simulink model "Mob_Cob_sim"  (R2023b)
settings: Solver=VariableStepAuto  StartTime=0.0  StopTime=5  MinStep=1e-5  RelTol=1e-2
values from neighbouring files (symbols this model uses):
  Mob_Cob = SerialLink(links,'name','Mobile_Cobot')    [Mob_Cob_plots.m]    (also in Omron_Mob_Cob.m; Omron_Mobile_Cobot.m; Updated_SCM_mobile_cobot_kinematics_no_dummy_frames.m; testing.m)
  q1 = ones(1,9)    [testing.m]
  q2 = ones(1,27)    [testing.m]
undefined symbols (not defined in the file or in its folder): coriolis, p560
libraries: roblocks x8
settings Model: Creator=jehuy  LastModifiedBy=kangwang

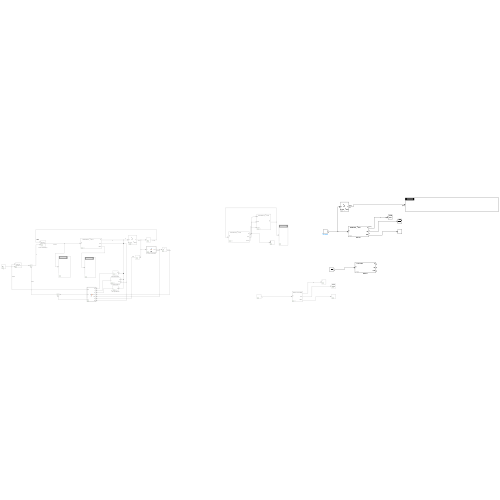
[thumbnail: Simulink's stored preview of the top-level diagram]
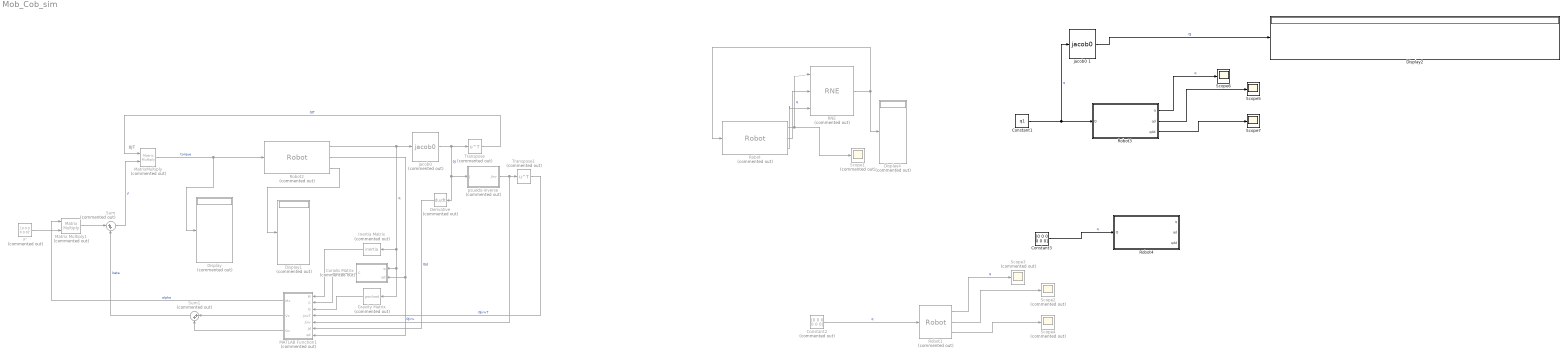
== system Mob_Cob_sim ==
  note: 0JT
  Constant1 : Constant  Value=q1
  Constant2 : Constant  Commented=on  Value=[0 0 0 0 0 0]
  Constant3 : Constant  Value=[0 0 0 0 0 0]
  Coriolis Matrix : Subsystem  Commented=on  mask{robot=Mob_Cob}
  Derivative : Derivative  Commented=on
  Display : Display  Commented=on
  Display1 : Display  Commented=on
  Display2 : Display
  Display4 : Display  Commented=on
  F' : Constant  Commented=on  Value=[0 0 0 0 0 0]'
  Gravity Matrix : roblocks/Arm/gravload  Commented=on  robot=Mob_Cob
  Inertia Matrix : roblocks/Arm/inertia  Commented=on  robot=Mob_Cob
  MATLAB Function1 : MATLAB Function  Commented=on  TreatAsAtomicUnit=on
  Matrix Multiply1 : Product  Commented=on  Multiplication=Matrix(*)
  MatrixMultiply : Product  Commented=on  Multiplication=Matrix(*)
  RNE : roblocks/Arm/RNE  Commented=on  robot=Mob_Cob.nofriction  grav=[0 0 9.81]
  Robot : roblocks/Arm/Robot  Commented=on  robot=Mob_Cob.nofriction  q0=[1 1 1 1 1 1 1 1 1]
      link override Integrator: InitialCondition=0
      link override Integrator1: InitialCondition=[1 1 1 1 1 1 1 1 1]
      link override S-Function: Parameters=robot
  Robot1 : roblocks/Arm/Robot  Commented=on  robot=p560.nofriction  q0=[0 0 0 0 0 0]
      link override Integrator1: InitialCondition=[0 0 0 0 0 0]
  Robot2 : roblocks/Arm/Robot  Commented=on  robot=Mob_Cob.nofriction  q0=[1 1 1 1 1 1 1 1 1]
      link override Integrator: InitialCondition=0
      link override Integrator1: InitialCondition=[1 1 1 1 1 1 1 1 1]
      link override S-Function: Parameters=robot
  Robot3 : Subsystem  AncestorBlock=roblocks/Arm/Robot  mask{robot=Mob_Cob.nofriction, q0=q1}
      mask prompts: robot "Robot object"; q0 "Initial state"
      mask help: Rigid-body dynamic model of robot.
      mask init:
      | if isa(robot, 'SerialLink')
      |     rname = robot.name;
      |     %fprintf('**robot name is %s\n', rname);
      | else
      |     rname = '';
      |     n = 0
      | end
      mask Help:
      | Simulates the forward (direct) rigid-body dynamics of the robot described
      | by the given robot object.  For given applied joint torque/force it computes
      | the instaneous joint coordinates, velocities and acclerations.
      | 
      | 
      | <b>Parameters::</b>
      | 
      | robot (SerialLink) a dynamic model of an N-link serial link manipulator
      | q0 (1xN)  Initial joint coordinates
      | 
      | <b>Inputs::</b>
      | 
      | Q (1xN) the generalized joint force (torque or force) required to achieve
      | the motion state (q, qd, qdd).
      | 
      | <b>Outputs::</b>
      | 
      | q (1xN) joint coordinates
      | qd (1xN) joint coordinate velocity
      | qdd (1xN) joint coordinate acceleration
      | 
      | 
      | <b>Notes::</b>
      | 
      | - Required to simulate robot rigid body motion.
      | - Implemented using the recursive Newton-Euler scheme (RNE).
      | - A wrapper for the Toolbox method accel() which in turn depends on the
      |   method rne().
      mask Display:
      | port_label('input', 1, 'Q')
      | port_label('output', 1, 'q')
      | port_label('output', 2, 'qd')
      | port_label('output', 3, 'qdd')
      | text(0.1, 0.9,  rname, 'horizontalAlignment', 'left')
  Robot4 : Subsystem  AncestorBlock=roblocks/Arm/Robot  mask{robot=p560, q0=q1}
      mask prompts: robot "Robot object"; q0 "Initial state"
      mask help: Rigid-body dynamic model of robot.
      mask init:
      | if isa(robot, 'SerialLink')
      |     rname = robot.name;
      |     %fprintf('**robot name is %s\n', rname);
      | else
      |     rname = '';
      |     n = 0
      | end
      mask Help:
      | Simulates the forward (direct) rigid-body dynamics of the robot described
      | by the given robot object.  For given applied joint torque/force it computes
      | the instaneous joint coordinates, velocities and acclerations.
      | 
      | 
      | <b>Parameters::</b>
      | 
      | robot (SerialLink) a dynamic model of an N-link serial link manipulator
      | q0 (1xN)  Initial joint coordinates
      | 
      | <b>Inputs::</b>
      | 
      | Q (1xN) the generalized joint force (torque or force) required to achieve
      | the motion state (q, qd, qdd).
      | 
      | <b>Outputs::</b>
      | 
      | q (1xN) joint coordinates
      | qd (1xN) joint coordinate velocity
      | qdd (1xN) joint coordinate acceleration
      | 
      | 
      | <b>Notes::</b>
      | 
      | - Required to simulate robot rigid body motion.
      | - Implemented using the recursive Newton-Euler scheme (RNE).
      | - A wrapper for the Toolbox method accel() which in turn depends on the
      |   method rne().
      mask Display:
      | port_label('input', 1, 'Q')
      | port_label('output', 1, 'q')
      | port_label('output', 2, 'qd')
      | port_label('output', 3, 'qdd')
      | text(0.1, 0.9,  rname, 'horizontalAlignment', 'left')
  Scope{1..4} (4 alike) : Scope  Commented=on
  Scope5 : Scope
  Scope6 : Scope
  Scope7 : Scope
  Sum : Sum  Commented=on  Inputs=|++
  Sum1 : Sum  Commented=on  Inputs=|++
  Transpose : Math  Commented=on  Operator=transpose
  Transpose1 : Math  Commented=on  Operator=transpose
  "jacob0 " : roblocks/Arm/jacob0   Commented=on  robot=Mob_Cob
  jacob0 1 : roblocks/Arm/jacob0   robot=Mob_Cob
  psuedo-inverse : MATLAB Function  Commented=on  TreatAsAtomicUnit=on
  wires:
  "jacob0 "/1 -> psuedo-inverse/1(J), Derivative/1, Transpose/1  "0J"
  psuedo-inverse/1(Jinv) -> MATLAB Function1/5(Jinv), Transpose1/1  "0Jinv"
  Transpose1/1 -> MATLAB Function1/4(JinvT)  "0JinvT"
  Transpose/1 -> MatrixMultiply/1  "0JT"
  Inertia Matrix/1 -> MATLAB Function1/1(M)
  Coriolis Matrix/1(C) -> MATLAB Function1/2(C)
  Derivative/1 -> MATLAB Function1/6(Jd)  "0Jd"
  MATLAB Function1/2(Vx) -> Sum1/1
  MATLAB Function1/3(Gx) -> Sum1/2
  Gravity Matrix/1 -> MATLAB Function1/3(G)
  Robot2/1 -> Gravity Matrix/1, Coriolis Matrix/1(q), Inertia Matrix/1, "jacob0 "/1  "q"
  F'/1 -> Matrix Multiply1/2
  MATLAB Function1/1(Mx) -> Matrix Multiply1/1  "alpha"
  Matrix Multiply1/1 -> Sum/1
  Sum1/1 -> Sum/2  "beta"
  Sum/1 -> MatrixMultiply/2  "F"
  MatrixMultiply/1 -> Robot2/1, Display/1  "torque"
  Constant2/1 -> Robot1/1  "q"
  Robot1/2 -> Scope2/1
  Robot1/1 -> Scope3/1  "q"
  Robot1/3 -> Scope4/1
  Robot/1 -> RNE/1, Scope1/1  "q"
  Robot2/2 -> MATLAB Function1/7(qd), Coriolis Matrix/2(qd)
  Robot2/3 -> Display1/1
  Robot/3 -> RNE/3
  Robot/2 -> RNE/2
  RNE/1 -> Display4/1, Robot/1
  Constant1/1 -> jacob0 1/1, Robot3/1(Q)  "q"
  Robot3/1(q) -> Scope6/1  "q"
  Robot3/2(qd) -> Scope5/1
  Robot3/3(qdd) -> Scope7/1
  jacob0 1/1 -> Display2/1  "0J"
  Constant3/1 -> Robot4/1(Q)  "q"

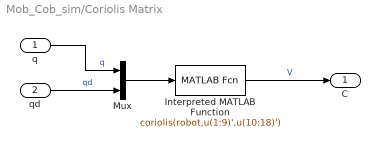
== system Mob_Cob_sim/Coriolis Matrix ==
  q : Inport
  qd : Inport  Port=2
  Interpreted MATLAB Function : MATLABFcn  MATLABFcn=coriolis(robot,u(1:9)',u(10:18)')  Output1D=off
  Mux : Mux  Inputs=2
  C : Outport
  wires:
  Mux/1 -> Interpreted MATLAB Function/1
  q/1 -> Mux/1  "q"
  qd/1 -> Mux/2  "qd"
  Interpreted MATLAB Function/1 -> C/1  "V"

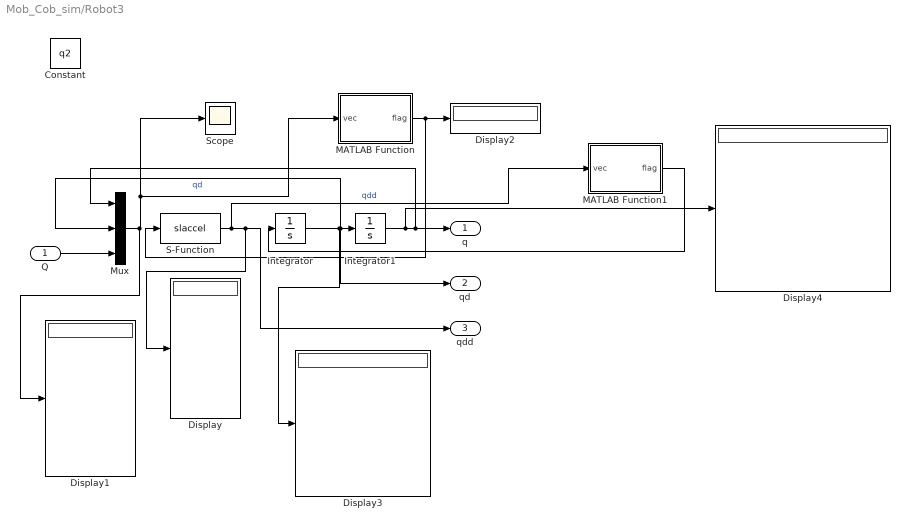
== system Mob_Cob_sim/Robot3 ==
  Q : Inport
  Constant : Constant  Value=q2
  Display{,1..4} (5 alike) : Display
  Integrator : Integrator
  Integrator1 : Integrator  InitialCondition=q1
  MATLAB Function : MATLAB Function  TreatAsAtomicUnit=on
  MATLAB Function1 : MATLAB Function  TreatAsAtomicUnit=on
  Mux : Mux  Inputs=3
  S-Function : S-Function  FunctionName=slaccel  Parameters=robot  SFunctionDeploymentMode=off  EnableBusSupport=off
  Scope : Scope
  q : Outport  VectorParamsAs1DForOutWhenUnconnected=off
  qd : Outport  Port=2  VectorParamsAs1DForOutWhenUnconnected=off
  qdd : Outport  Port=3  VectorParamsAs1DForOutWhenUnconnected=off
  wires:
  S-Function/1 -> MATLAB Function1/1(vec), Display/1, qdd/1  "qdd"
  Mux/1 -> Display1/1, Scope/1, MATLAB Function/1(vec)
  Integrator/1 -> Display3/1, qd/1, Integrator1/1, Mux/2  "qd"
  Q/1 -> Mux/3
  Integrator1/1 -> Display4/1, q/1, Mux/1
  MATLAB Function/1(flag) -> S-Function/1, Display2/1
  MATLAB Function1/1(flag) -> Integrator/1

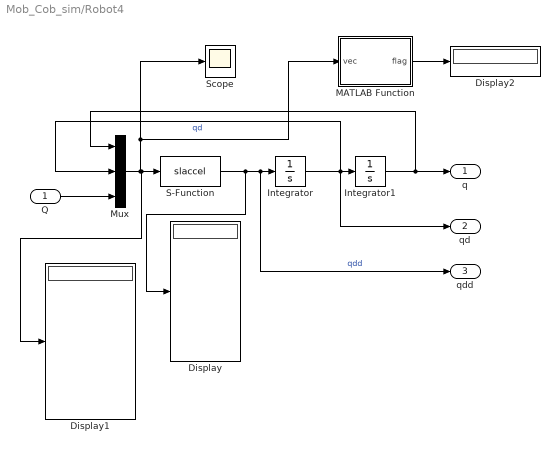
== system Mob_Cob_sim/Robot4 ==
  Q : Inport
  Display : Display
  Display1 : Display
  Display2 : Display
  Integrator : Integrator
  Integrator1 : Integrator
  MATLAB Function : MATLAB Function  TreatAsAtomicUnit=on
  Mux : Mux  Inputs=3
  S-Function : S-Function  FunctionName=slaccel  Parameters=robot  SFunctionDeploymentMode=off  EnableBusSupport=off
  Scope : Scope
  q : Outport  VectorParamsAs1DForOutWhenUnconnected=off
  qd : Outport  Port=2  VectorParamsAs1DForOutWhenUnconnected=off
  qdd : Outport  Port=3  VectorParamsAs1DForOutWhenUnconnected=off
  wires:
  S-Function/1 -> Display/1, qdd/1, Integrator/1  "qdd"
  Mux/1 -> Scope/1, MATLAB Function/1(vec), Display1/1, S-Function/1
  Integrator/1 -> qd/1, Integrator1/1, Mux/2  "qd"
  Q/1 -> Mux/3
  Integrator1/1 -> q/1, Mux/1
  MATLAB Function/1(flag) -> Display2/1

== matlab function Mob_Cob_sim/MATLAB Function1 ==
  data: M input; Mx output; C input; G input; JinvT input; Jinv input; Jd input; qd input; Vx output; Gx output
function [Mx,Vx,Gx]= fcn(M,C,G,JinvT,Jinv,Jd,qd)

V=C*qd;

Mx=JinvT*M*Jinv;
Gx=JinvT*G';
Vx=JinvT*(V-M*Jinv*Jd*qd);

== matlab function Mob_Cob_sim/Robot3/MATLAB Function ==
  data: vec input; flag output
function flag = checkVals(vec)
display(vec)
if any(isnan(vec)) || any(isinf(vec))
        flag = ones(27,1)
    else
        flag = vec
    end
end

== matlab function Mob_Cob_sim/psuedo-inverse ==
  data: J input; Jinv output
function Jinv = fcn(J)

Jinv = pinv(J);

== matlab function Mob_Cob_sim/Robot4/MATLAB Function ==
  data: vec input; flag output
function flag = checkVals(vec)
    if any(isnan(vec)) || any(isinf(vec))
        flag = -1;
    else
        flag = 1;
    end
end

== matlab function Mob_Cob_sim/Robot3/MATLAB Function1 ==
  data: vec input; flag output
function flag = checkVals(vec)
display(vec)
if any(isnan(vec)) || any(isinf(vec))
        flag = [1,1,1,1,1,1,1,1,1].'
    else
        flag = vec
    end
end
